simulink model "dcm2att"  (R2018a)
settings: Solver=VariableStepAuto  StartTime=0.0  StopTime=10.0  RelTol=1e-3
settings Model: Creator=lamy  LastModifiedBy=lamy

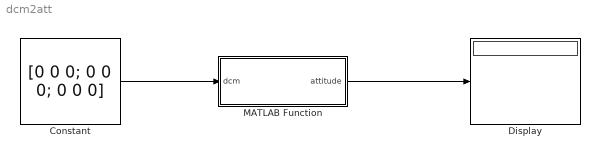
== system dcm2att ==
  Constant : Constant  Value=[0 0 0; 0 0 0; 0 0 0]
  Display : Display
  MATLAB Function : MATLAB Function  TreatAsAtomicUnit=on
  wires:
  Constant/1 -> MATLAB Function/1(dcm)
  MATLAB Function/1(attitude) -> Display/1

== matlab function dcm2att/MATLAB Function ==
  data: dcm input; attitude output
function attitude = dcm2att(dcm)
yaw = atan2(dcm(1,2), dcm(1,1));
pitch = -asin(dcm(1,3));
roll = atan2(dcm(2,3),dcm(3,3));
attitude = [roll; pitch; yaw];
